simulink model "two_cycle_normal"  (R2023b)
settings: Solver=ode45  StartTime=0.0  StopTime=12  RelTol=1e-3
values from neighbouring files (symbols this model uses):
  Cv = 36    [av_debug.m]
  Emax1 = 3    [av_debug.m]
  HR = 80    [av_debug.m]
  Rscr = 1.1    [av_debug.m]
undefined symbols (not defined in the file or in its folder): Ca
settings Model: Creator=19908  LastModifiedBy=19908

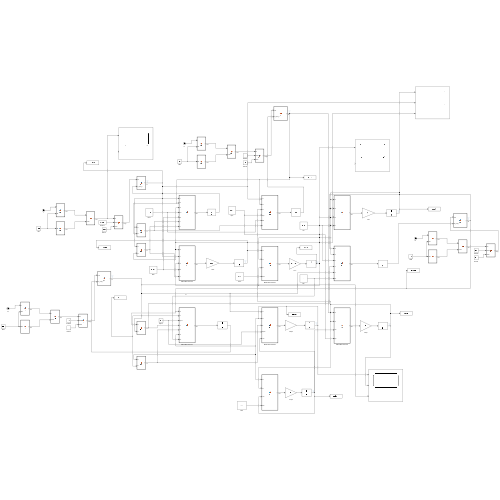
[thumbnail: Simulink's stored preview of the top-level diagram]
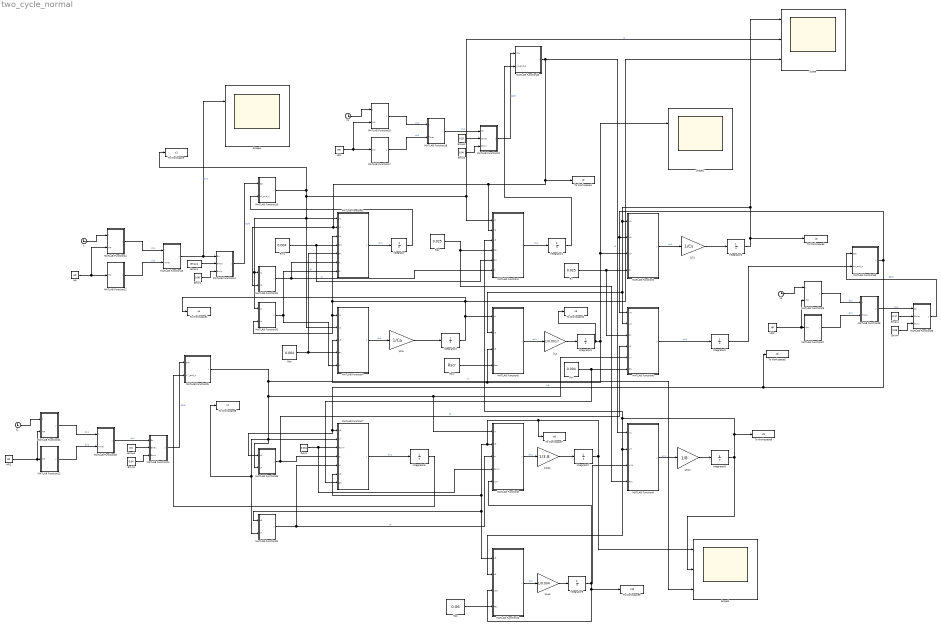
== system two_cycle_normal ==
  1/CA : Gain  Gain=1/Ca
  1/CpA : Gain  Gain=1/3.8
  1/Cpv : Gain  Gain=1/8
  1/Cv : Gain  Gain=1/Cv
  1/LpA : Gain  Gain=1/0.034
  1/Ls : Gain  Gain=1/0.0017
  Emax1 : Constant  Value=Emax1
  Emax2 : Constant  Value=0.15
  Emax3 : Constant  Value=0.6
  Emax4 : Constant  Value=0.17
  Emin1 : Constant  Value=0.08
  Emin2 : Constant  Value=0.04
  Emin3 : Constant  Value=0.04
  Emin4 : Constant  Value=0.08
  HR{,1..3} (4 alike) : Constant  Value=HR
  Integrator : Integrator  InitialCondition=125
  Integrator1 : Integrator  InitialCondition=150
  Integrator2 : Integrator  InitialCondition=80
  Integrator3 : Integrator
  Integrator4 : Integrator  InitialCondition=6
  Integrator5 : Integrator  InitialCondition=50
  Integrator6 : Integrator  InitialCondition=325
  Integrator7 : Integrator  InitialCondition=12
  Integrator8 : Integrator  InitialCondition=8
  Integrator9 : Integrator
  MATLAB Function1 : MATLAB Function  TreatAsAtomicUnit=on
  MATLAB Function10 : MATLAB Function  TreatAsAtomicUnit=on
  MATLAB Function11 : MATLAB Function  TreatAsAtomicUnit=on
  MATLAB Function12 : MATLAB Function  TreatAsAtomicUnit=on
  MATLAB Function13 : MATLAB Function  TreatAsAtomicUnit=on
  MATLAB Function14 : MATLAB Function  TreatAsAtomicUnit=on
  MATLAB Function15 : MATLAB Function  TreatAsAtomicUnit=on
  MATLAB Function16 : MATLAB Function  TreatAsAtomicUnit=on
  MATLAB Function17 : MATLAB Function  TreatAsAtomicUnit=on
  MATLAB Function18 : MATLAB Function  TreatAsAtomicUnit=on
  MATLAB Function19 : MATLAB Function  TreatAsAtomicUnit=on
  MATLAB Function2 : MATLAB Function  TreatAsAtomicUnit=on
  MATLAB Function20 : MATLAB Function  TreatAsAtomicUnit=on
  MATLAB Function21 : MATLAB Function  TreatAsAtomicUnit=on
  MATLAB Function22 : MATLAB Function  TreatAsAtomicUnit=on
  MATLAB Function23 : MATLAB Function  TreatAsAtomicUnit=on
  MATLAB Function24 : MATLAB Function  TreatAsAtomicUnit=on
  MATLAB Function25 : MATLAB Function  TreatAsAtomicUnit=on
  MATLAB Function26 : MATLAB Function  TreatAsAtomicUnit=on
  MATLAB Function27 : MATLAB Function  TreatAsAtomicUnit=on
  MATLAB Function28 : MATLAB Function  TreatAsAtomicUnit=on
  MATLAB Function29 : MATLAB Function  TreatAsAtomicUnit=on
  MATLAB Function3 : MATLAB Function  TreatAsAtomicUnit=on
  MATLAB Function30 : MATLAB Function  TreatAsAtomicUnit=on
  MATLAB Function31 : MATLAB Function  TreatAsAtomicUnit=on
  MATLAB Function32 : MATLAB Function  TreatAsAtomicUnit=on
  MATLAB Function33 : MATLAB Function  TreatAsAtomicUnit=on
  MATLAB Function34 : MATLAB Function  TreatAsAtomicUnit=on
  MATLAB Function4 : MATLAB Function  TreatAsAtomicUnit=on
  MATLAB Function5 : MATLAB Function  TreatAsAtomicUnit=on
  MATLAB Function6 : MATLAB Function  TreatAsAtomicUnit=on
  MATLAB Function7 : MATLAB Function  TreatAsAtomicUnit=on
  MATLAB Function8 : MATLAB Function  TreatAsAtomicUnit=on
  MATLAB Function9 : MATLAB Function  TreatAsAtomicUnit=on
  Rac : Constant  Value=0.06
  Rav : Constant  Value=0.004
  Rmv : Constant  Value=0.004
  Rpv : Constant  Value=0.025
  Rpvm : Constant  Value=0.004
  Rscr : Constant  Value=Rscr
  Rtv : Constant  Value=0.004
  Rv : Constant  Value=0.025
  Scope : Scope  NumInputPorts=3
  Scope1 : Scope  NumInputPorts=3
  Scope2 : Scope  NumInputPorts=2
  Scope3 : Scope  NumInputPorts=2
  To Workspace : ToWorkspace  VariableName=x1  SaveFormat=Timeseries  SampleTime=-1
  To Workspace1 : ToWorkspace  VariableName=x4  SaveFormat=Timeseries  SampleTime=-1
  To Workspace2 : ToWorkspace  VariableName=x5  SaveFormat=Timeseries  SampleTime=-1
  To Workspace3 : ToWorkspace  VariableName=x3  SaveFormat=Timeseries  SampleTime=-1
  To Workspace4 : ToWorkspace  VariableName=x2  SaveFormat=Timeseries  SampleTime=-1
  To Workspace5 : ToWorkspace  VariableName=x6  SaveFormat=Timeseries  SampleTime=-1
  To Workspace6 : ToWorkspace  VariableName=x7  SaveFormat=Timeseries  SampleTime=-1
  To Workspace7 : ToWorkspace  VariableName=x8  SaveFormat=Timeseries  SampleTime=-1
  To Workspace8 : ToWorkspace  VariableName=x9  SaveFormat=Timeseries  SampleTime=-1
  To Workspace9 : ToWorkspace  VariableName=x10  SaveFormat=Timeseries  SampleTime=-1
  t{,1..3} (4 alike) : Clock
  wires:
  MATLAB Function1/1(y) -> Integrator/1  "dx1"
  MATLAB Function2/1(y) -> Integrator1/1  "dx1"
  MATLAB Function9/1(y) -> 1/Cpv/1  "dx1"
  1/Cpv/1 -> Integrator8/1
  Integrator8/1 -> Scope1/2, MATLAB Function2/3(x9), MATLAB Function10/2(x9), MATLAB Function9/2(x9), To Workspace8/1
  MATLAB Function8/1(y) -> 1/CpA/1  "dx1"
  1/CpA/1 -> Integrator7/1
  Integrator7/1 -> Scope1/1, To Workspace7/1, MATLAB Function7/6(x8), MATLAB Function34/1(x8), MATLAB Function10/1(x8), MATLAB Function8/2(x8)
  MATLAB Function7/1(y) -> Integrator6/1  "dx1"
  MATLAB Function3/1(y) -> 1/Cv/1  "dx1"
  1/Cv/1 -> Integrator4/1
  Integrator4/1 -> Scope/1, MATLAB Function5/2(x3), MATLAB Function6/2(x3), MATLAB Function3/1(x3), To Workspace3/1
  MATLAB Function6/1(y) -> Integrator5/1  "dx1"
  MATLAB Function5/1(y) -> 1/Ls/1  "dx1"
  1/Ls/1 -> Integrator3/1
  Integrator3/1 -> To Workspace2/1, Scope2/1, MATLAB Function3/3(x5), MATLAB Function5/3(x5), MATLAB Function4/3(x5)
  1/CA/1 -> Integrator2/1
  MATLAB Function4/1(y) -> 1/CA/1  "dx1"
  Integrator2/1 -> MATLAB Function5/1(x4), To Workspace1/1, MATLAB Function1/3(x4), MATLAB Function32/2(x4), MATLAB Function4/1(x4), Scope/3
  MATLAB Function10/1(y) -> 1/LpA/1  "dx1"
  1/LpA/1 -> Integrator9/1
  Integrator9/1 -> MATLAB Function8/5(x10), MATLAB Function9/3(x10), To Workspace9/1, MATLAB Function10/3(x10)
  Rac/1 -> MATLAB Function10/4(Rac)
  Rscr/1 -> MATLAB Function5/4(Rscr)
  Rav/1 -> MATLAB Function1/5(RA), MATLAB Function4/4(RA)
  Rmv/1 -> MATLAB Function2/5(Rm), MATLAB Function1/4(Rm)
  Rpv/1 -> MATLAB Function9/4(Rpv), MATLAB Function2/4(Rpv)
  Rv/1 -> MATLAB Function6/3(Rv), MATLAB Function3/4(Rv)
  Rtv/1 -> MATLAB Function7/7(Rtv), MATLAB Function6/6(Rtv)
  Rpvm/1 -> MATLAB Function8/4(Rpvm), MATLAB Function7/3(Rpvm)
  t/1 -> MATLAB Function11/1(t)
  HR/1 -> MATLAB Function11/2(HR), MATLAB Function12/1(HR)
  MATLAB Function11/1(y) -> MATLAB Function13/1(t)  "dx1"
  MATLAB Function12/1(y) -> MATLAB Function13/2(Tmax)  "dx1"
  MATLAB Function13/1(y) -> Scope3/1, MATLAB Function14/1(En)  "dx1"
  Emax1/1 -> MATLAB Function14/2(Emax)
  Emin1/1 -> MATLAB Function14/3(Emin)
  MATLAB Function14/1(y) -> MATLAB Function15/1(C1t)  "C1(t)"
  Integrator/1 -> MATLAB Function15/2(x1_and_c)
  MATLAB Function15/1(y) -> To Workspace/1, MATLAB Function4/2(x1), MATLAB Function32/1(x1), MATLAB Function31/1(x1), MATLAB Function1/1(x1), Scope/2, MATLAB Function2/1(x1)  "x1"
  t1/1 -> MATLAB Function16/1(t)
  MATLAB Function17/1(y) -> MATLAB Function18/2(Tmax)  "dx1"
  MATLAB Function19/1(y) -> MATLAB Function20/1(C2t)  "C2(t)"
  MATLAB Function16/1(y) -> MATLAB Function18/1(t)  "dx1"
  MATLAB Function18/1(y) -> MATLAB Function19/1(En)  "dx1"
  HR1/1 -> MATLAB Function16/2(HR), MATLAB Function17/1(HR)
  Emax2/1 -> MATLAB Function19/2(Emax)
  Emin2/1 -> MATLAB Function19/3(Emin)
  Integrator1/1 -> MATLAB Function20/2(x2_and_c)
  MATLAB Function20/1(y) -> To Workspace4/1, MATLAB Function31/2(x2), MATLAB Function1/2(x2), MATLAB Function2/2(x2), MATLAB Function9/1(x2)  "x2"
  MATLAB Function23/1(y) -> MATLAB Function24/1(En)  "dx1"
  HR2/1 -> MATLAB Function21/2(HR), MATLAB Function22/1(HR)
  Emax3/1 -> MATLAB Function24/2(Emax)
  MATLAB Function24/1(y) -> MATLAB Function25/1(C4t)  "C4(t)"
  t2/1 -> MATLAB Function21/1(t)
  MATLAB Function22/1(y) -> MATLAB Function23/2(Tmax)  "dx1"
  Emin3/1 -> MATLAB Function24/3(Emin)
  Integrator6/1 -> MATLAB Function25/2(x7_and_c)
  MATLAB Function21/1(y) -> MATLAB Function23/1(t)  "dx1"
  MATLAB Function25/1(y) -> Scope1/3, MATLAB Function8/1(x7), MATLAB Function6/5(x7), To Workspace6/1, MATLAB Function34/2(x7), MATLAB Function33/2(x7), MATLAB Function7/2(x7)  "x7"
  MATLAB Function28/1(y) -> MATLAB Function29/1(En)  "dx1"
  HR3/1 -> MATLAB Function26/2(HR), MATLAB Function27/1(HR)
  Emax4/1 -> MATLAB Function29/2(Emax)
  MATLAB Function29/1(y) -> MATLAB Function30/1(C3t)  "C3(t)"
  t3/1 -> MATLAB Function26/1(t)
  MATLAB Function27/1(y) -> MATLAB Function28/2(Tmax)  "dx1"
  Emin4/1 -> MATLAB Function29/3(Emin)
  MATLAB Function26/1(y) -> MATLAB Function28/1(t)  "dx1"
  Integrator5/1 -> MATLAB Function30/2(x6_and_c)
  MATLAB Function30/1(y) -> To Workspace5/1, MATLAB Function33/1(x6), MATLAB Function7/1(x6), MATLAB Function3/2(x6), MATLAB Function6/1(x6)  "x6"
  MATLAB Function31/1(y) -> MATLAB Function2/6(r1), MATLAB Function1/6(r1)  "r1"
  MATLAB Function32/1(y) -> MATLAB Function4/5(r2), MATLAB Function1/7(r2)  "r2"
  MATLAB Function33/1(y) -> MATLAB Function6/4(r3), MATLAB Function7/4(r3)  "r3"
  MATLAB Function34/1(y) -> MATLAB Function8/3(r4), MATLAB Function7/5(r4)  "r4"

== matlab function two_cycle_normal/MATLAB Function8 ==
  data: x7 input; x8 input; r4 input; Rpvm input; y output; x10 input
function y = fcn(x7,x8,r4,Rpvm,x10)
y=-r4*(x8-x7)/Rpvm-x10;

== matlab function two_cycle_normal/MATLAB Function9 ==
  data: x2 input; x9 input; x10 input; Rpv input; y output
function y = fcn(x2,x9,x10,Rpv)
y=x10-(x9-x2)/Rpv;

== matlab function two_cycle_normal/MATLAB Function10 ==
  data: x8 input; x9 input; x10 input; Rac input; y output
function y = fcn(x8,x9,x10,Rac)
y=x8-x9-x10*Rac;

== matlab function two_cycle_normal/MATLAB Function11 ==
  data: y output; t input; HR input
function y = fcn(t,HR)
y=rem(t,60/HR);

== matlab function two_cycle_normal/MATLAB Function12 ==
  data: y output; HR input
function y = fcn(HR)
y=0.2+0.05*60/HR;

== matlab function two_cycle_normal/MATLAB Function13 ==
  data: y output; t input; Tmax input
function y = fcn(t,Tmax)
tn=t/Tmax;
a=(tn/0.7)^1.9;
b=(tn/1.17)^21.9;
y=1.55*(a/(1+a))*(1/(1+b));

== matlab function two_cycle_normal/MATLAB Function14 ==
  data: y output; En input; Emax input; Emin input
function y = fcn(En,Emax,Emin)
E=(Emax-Emin)*En+Emin;
y=1/E;

== matlab function two_cycle_normal/MATLAB Function15 ==
  data: y output; C1t input; x1_and_c input
function y = fcn(C1t,x1_and_c)
y=x1_and_c/C1t;

== matlab function two_cycle_normal/MATLAB Function16 ==
  data: y output; t input; HR input
function y = fcn(t,HR)
y=rem(t,60/HR);

== matlab function two_cycle_normal/MATLAB Function17 ==
  data: y output; HR input
function y = fcn(HR)
y=0.2+0.05*60/HR;

== matlab function two_cycle_normal/MATLAB Function18 ==
  data: y output; t input; Tmax input
function y = fcn(t,Tmax)
tn=t/Tmax;
a=(tn/0.7)^1.9;
b=(tn/1.17)^21.9;
y=1.55*(a/(1+a))*(1/(1+b));

== matlab function two_cycle_normal/MATLAB Function19 ==
  data: y output; En input; Emax input; Emin input
function y = fcn(En,Emax,Emin)
E=(Emax-Emin)*En+Emin;
y=1/E;

== matlab function two_cycle_normal/MATLAB Function2 ==
  data: y output; x1 input; x2 input; x9 input; Rpv input; Rm input; r1 input
function y = fcn(x1,x2,x9,Rpv,Rm,r1)
y=(x9-x2)/(Rpv)-r1*(x2-x1)/Rm;

== matlab function two_cycle_normal/MATLAB Function20 ==
  data: y output; C2t input; x2_and_c input
function y = fcn(C2t,x2_and_c)
y=x2_and_c/C2t;

== matlab function two_cycle_normal/MATLAB Function21 ==
  data: y output; t input; HR input
function y = fcn(t,HR)
y=rem(t,60/HR);

== matlab function two_cycle_normal/MATLAB Function22 ==
  data: y output; HR input
function y = fcn(HR)
y=0.2+0.05*60/HR;

== matlab function two_cycle_normal/MATLAB Function23 ==
  data: y output; t input; Tmax input
function y = fcn(t,Tmax)
tn=t/Tmax;
a=(tn/0.7)^1.9;
b=(tn/1.17)^21.9;
y=1.55*(a/(1+a))*(1/(1+b));

== matlab function two_cycle_normal/MATLAB Function24 ==
  data: y output; En input; Emax input; Emin input
function y = fcn(En,Emax,Emin)
E=(Emax-Emin)*En+Emin;
y=1/E;

== matlab function two_cycle_normal/MATLAB Function25 ==
  data: y output; C4t input; x7_and_c input
function y = fcn(C4t,x7_and_c)
y=x7_and_c/C4t;

== matlab function two_cycle_normal/MATLAB Function26 ==
  data: y output; t input; HR input
function y = fcn(t,HR)
y=rem(t,60/HR);

== matlab function two_cycle_normal/MATLAB Function27 ==
  data: y output; HR input
function y = fcn(HR)
y=0.2+0.05*60/HR;

== matlab function two_cycle_normal/MATLAB Function28 ==
  data: y output; t input; Tmax input
function y = fcn(t,Tmax)
tn=t/Tmax;
a=(tn/0.7)^1.9;
b=(tn/1.17)^21.9;
y=1.55*(a/(1+a))*(1/(1+b));

== matlab function two_cycle_normal/MATLAB Function29 ==
  data: y output; En input; Emax input; Emin input
function y = fcn(En,Emax,Emin)
E=(Emax-Emin)*En+Emin;
y=1/E;

== matlab function two_cycle_normal/MATLAB Function30 ==
  data: y output; C3t input; x6_and_c input
function y = fcn(C3t,x6_and_c)
y=x6_and_c/C3t;

== matlab function two_cycle_normal/MATLAB Function31 ==
  data: y output; x1 input; x2 input
function y = fcn(x1,x2)
if x2>=x1
    y=1;
else 
    y=0;
end

== matlab function two_cycle_normal/MATLAB Function32 ==
  data: y output; x1 input; x4 input
function y = fcn(x1,x4)
if x1>=x4
    y=1;
else 
    y=0;
end

== matlab function two_cycle_normal/MATLAB Function33 ==
  data: y output; x6 input; x7 input
function y = fcn(x6,x7)
if x6>=x7
    y=1;
else 
    y=0;
end

== matlab function two_cycle_normal/MATLAB Function34 ==
  data: y output; x8 input; x7 input
function y = fcn(x8,x7)
if x7>=x8
    y=1;
else 
    y=0;
end

== matlab function two_cycle_normal/MATLAB Function3 ==
  data: y output; x3 input; x6 input; x5 input; Rv input
function y = fcn(x3,x6,x5,Rv)
y=(x6-x3)/Rv+x5;

== matlab function two_cycle_normal/MATLAB Function4 ==
  data: y output; x4 input; x1 input; x5 input; RA input; r2 input
function y = fcn(x4,x1,x5,RA,r2)
y=r2*(x1-x4)/RA-x5;

== matlab function two_cycle_normal/MATLAB Function5 ==
  data: y output; x4 input; x3 input; x5 input; Rscr input
function y = fcn(x4,x3,x5,Rscr)
y=x4-x3-x5*Rscr;

== matlab function two_cycle_normal/MATLAB Function6 ==
  data: y output; x6 input; x3 input; Rv input; r3 input; x7 input; Rtv input
function y = fcn(x6,x3,Rv,r3,x7,Rtv)
y=(x3-x6)/Rv+r3*(x7-x6)/Rtv;

== matlab function two_cycle_normal/MATLAB Function1 ==
  data: y output; x1 input; x2 input; x4 input; Rm input; RA input; r1 input; r2 input
function y = fcn(x1,x2,x4,Rm,RA,r1,r2)
y=r1*(x2-x1)/(Rm)-r2*(x1-x4)/(RA);

== matlab function two_cycle_normal/MATLAB Function7 ==
  data: y output; x6 input; x7 input; Rpvm input; r3 input; r4 input; x8 input; Rtv input
function y = fcn(x6,x7,Rpvm,r3,r4,x8,Rtv)
y=r4*(x8-x7)/Rpvm-r3*(x7-x6)/Rtv;
